simulink model "Simulazione_COMPENSATORI"  (R2022b)
settings: Solver=VariableStepAuto  StartTime=0.0  StopTime=100  RelTol=1e-3
values from neighbouring files (symbols this model uses):
  A = [ 0    0     1     0 ... (first row only)    [Tirocinio4_main.m]
  A_d = A'    [ProgettoOsservatoreOTTIMO.m]    (also in Tirocinio4_main.m = [ 0    0     1     0)
  Ac_1 = A-(V*C)+(B*F)-(V*D*F)    [Tirocinio4_main.m]
  Ac_2 = [As mat;Bm*Cs Am]    [Tirocinio4_main.m]
  B = [0 0 1/m1 0 ]'    [Tirocinio4_main.m]
  B_d = C'    [ProgettoOsservatoreOTTIMO.m]    (also in Tirocinio4_main.m = [0 0 1/m1_d 0 ]')
  Bc_1 = V    [Tirocinio4_main.m]
  Bc_2 = [Bs;Bm*Ds]    [Tirocinio4_main.m]
  C = [1 0 0 0]    [Tirocinio4_main.m]
  C_d = [1 0 0 0]    [Tirocinio4_main.m]
  Cc_1 = -F    [Tirocinio4_main.m]
  Cc_2 = [Dm*Cs Cm]    [Tirocinio4_main.m]
  D = 0    [Tirocinio4_main.m]
  Dc_2 = Dm*Ds    (= 0)    [Tirocinio4_main.m]
  f = 1    [Tirocinio4_main.m]
  M = 1    [Tirocinio4_main.m]
  M0 = 3    [Tirocinio4_main.m]
  M1 = 2    [Tirocinio4_main.m]
  OM = 1.5    [Tirocinio4_main.m]
  x0 = [x1; x2; v1 ; v2 ]    [Tirocinio4_main.m]
libraries: simulink x3
settings Model: Creator=Danilo  LastModifiedBy=Danilo

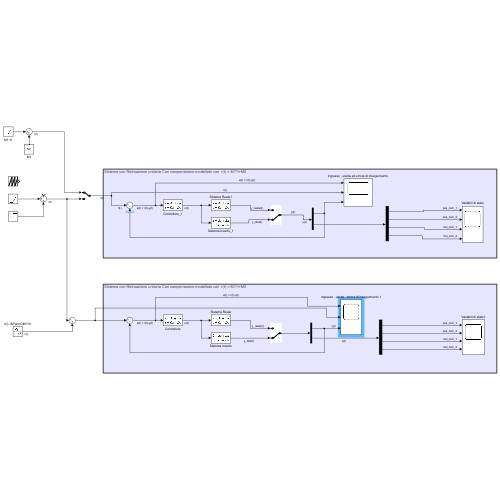
[thumbnail: Simulink's stored preview of the top-level diagram]
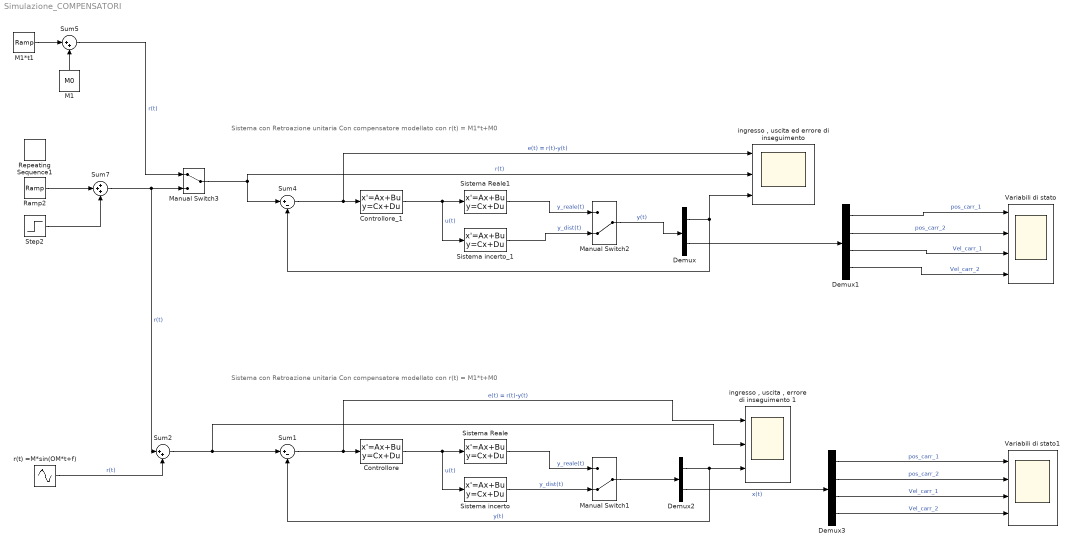
== system Simulazione_COMPENSATORI ==
  note: Sistema con Retroazione unitaria Con compensatore modellato con r(t) = M1*t+M0
  note: Sistema con Retroazione unitaria Con compensatore modellato con r(t) = M1*t+M0
  " r(t) =M*sin(OM*t+f) " : Sin  Amplitude=M  Frequency=OM  Phase=f  SampleTime=0
  Controllore : StateSpace  A=Ac_2  B=Bc_2  C=Cc_2  D=Dc_2  InitialCondition=0
  Controllore_1 : StateSpace  A=Ac_1  B=Bc_1  C=Cc_1  D=D  InitialCondition=0
  Demux : Demux  Outputs=2
  Demux1 : Demux
  Demux2 : Demux  Outputs=2
  Demux3 : Demux
  M1 : Constant  Value=M0
  M1*t1 : simulink/Sources/Ramp  slope=M1  start=0  InitialOutput=0
  Manual Switch1 : ManualSwitch  CurrentSetting=0
  Manual Switch2 : ManualSwitch  CurrentSetting=0
  Manual Switch3 : ManualSwitch
  Ramp2 : simulink/Sources/Ramp  slope=1  start=0  InitialOutput=0
  Repeating Sequence1 : simulink/Sources/Repeating Sequence  rep_seq_t=[0 30]  rep_seq_y=[0 10]
  Sistema Reale : StateSpace  A=A  B=B  C=[C; eye(4)]  D=[D ; zeros(4,1)]  InitialCondition=x0
  Sistema Reale1 : StateSpace  A=A  B=B  C=[C; eye(4)]  D=[D ; zeros(4,1)]  InitialCondition=x0
  Sistema incerto : StateSpace  A=A_d  B=B_d  C=[C_d; eye(4)]  D=[D;zeros(4,1)]  InitialCondition=x0
  Sistema incerto_1 : StateSpace  A=A_d  B=B_d  C=[C_d; eye(4)]  D=[D;zeros(4,1)]  InitialCondition=x0
  Step2 : Step  After=10  SampleTime=0
  Sum1 : Sum  Inputs=|+-
  Sum2 : Sum  Inputs=|++
  Sum4 : Sum  Inputs=|+-
  Sum5 : Sum  Inputs=|++
  Sum7 : Sum  Inputs=+++
  Variabili di stato : Scope  NumInputPorts=4
  Variabili di stato1 : Scope  NumInputPorts=4
  "ingresso , uscita , errore di inseguimento 1" : Scope  NumInputPorts=3
  "ingresso , uscita ed errore di inseguimento " : Scope  NumInputPorts=3
  wires:
  M1*t1/1 -> Sum5/1
  Ramp2/1 -> Sum7/2
  Step2/1 -> Sum7/3
  Sum5/1 -> Manual Switch3/1  "r(t)"
  Sistema incerto_1/1 -> Manual Switch2/2  "y_dist(t)"
  Manual Switch2/1 -> Demux/1  "y(t)"
  Sistema Reale1/1 -> Manual Switch2/1  "y_reale(t)"
  M1/1 -> Sum5/2
  Controllore_1/1 -> Sistema incerto_1/1, Sistema Reale1/1  "u(t)"
  Manual Switch3/1 -> "ingresso , uscita ed errore di inseguimento "/2, Sum4/1  "r(t)"
  Sum4/1 -> Controllore_1/1, "ingresso , uscita ed errore di inseguimento "/1  "e(t) = r(t)-y(t)"
  Demux/1 -> Sum4/2, "ingresso , uscita ed errore di inseguimento "/3
  Demux/2 -> Demux1/1
  Demux1/1 -> Variabili di stato/1  "pos_carr_1"
  Demux1/2 -> Variabili di stato/2  "pos_carr_2"
  Demux1/4 -> Variabili di stato/4  "Vel_carr_2"
  Demux1/3 -> Variabili di stato/3  "Vel_carr_1"
  Controllore/1 -> Sistema incerto/1, Sistema Reale/1  "u(t)"
  Demux2/1 -> Sum1/2, "ingresso , uscita , errore di inseguimento 1"/3  "y(t)"
  Demux3/2 -> Variabili di stato1/2  "pos_carr_2"
  Manual Switch1/1 -> Demux2/1
  Demux3/3 -> Variabili di stato1/3  "Vel_carr_1"
  Demux3/4 -> Variabili di stato1/4  "Vel_carr_2"
  Sistema Reale/1 -> Manual Switch1/1  "y_reale(t)"
  Demux2/2 -> Demux3/1  "x(t)"
  Sistema incerto/1 -> Manual Switch1/2  "y_dist(t)"
  Sum7/1 -> Sum2/1, Manual Switch3/2  "r(t)"
  Demux3/1 -> Variabili di stato1/1  "pos_carr_1"
  Sum1/1 -> Controllore/1, "ingresso , uscita , errore di inseguimento 1"/1  "e(t) = r(t)-y(t)"
  " r(t) =M*sin(OM*t+f) "/1 -> Sum2/2  "r(t)"
  Sum2/1 -> "ingresso , uscita , errore di inseguimento 1"/2, Sum1/1
